simulink model "PLL_sim_a"  (R2020a)
settings: Solver=ode45  StartTime=0.0  StopTime=5  RelTol=1e-6  EnableMultiTasking=on
undefined symbols (not defined in the file): Cf, Kvco, R1, R2, Ts, VDD
libraries: msbPllFoundation x2
settings Model: Creator=nicolas  LastModifiedBy=svanico
settings SolverCC: SolverResetMethod=Robust
settings DataIOCC: LimitDataPoints=on  SaveFormat=Array  SignalLoggingSaveFormat=ModelDataLogs  ReturnWorkspaceOutputs=off
settings OptimizationCC: ExpressionDepthLimit=2147483647  LifeSpan=inf
settings DebuggingCC: UnderspecifiedInitializationDetection=Classic  MergeDetectMultiDrivingBlocksExec=none  SolverPrmCheckMsg=warning  FcnCallInpInsideContextMsg=warning  StateNameClashWarn=warning  SFUnexpectedBacktrackingDiag=warning  SFNoUnconditionalDefaultTransitionDiag=warning  SFExecutionAtInitializationDiag=none  ArithmeticOperatorsInVariantConditions=warning
settings HardwareCC: ProdBitPerPointer=32  ProdBitPerSizeT=32  ProdBitPerPtrDiffT=32  ProdLargestAtomicFloat=None  ProdIntDivRoundTo=Undefined  ProdEndianess=Unspecified  ProdWordSize=32  ProdHWDeviceType=32-bit Generic
settings ModelReferenceCC: EnableRefExpFcnMdlSchedulingChecks=off  PropagateSignalLabelsOutOfModel=off
settings SFSimCC: SimUseLocalCustomCode=off  CustomCodeUndefinedFunction=UseInterfaceOnly
settings RTWCC: RTWUseLocalCustomCode=off
settings CodeAppCC: StateflowObjectComments=on
settings GRTTargetCC: TargetLangStandard=C89/C90 (ANSI)  CombineOutputUpdateFcns=off  GRTInterface=on
settings ConfigComp: CovMetricSettings=dw  CovSaveCumulativeToWorkspaceVar=on  CovSaveSingleToWorkspaceVar=on  CovExternalEMLEnable=off

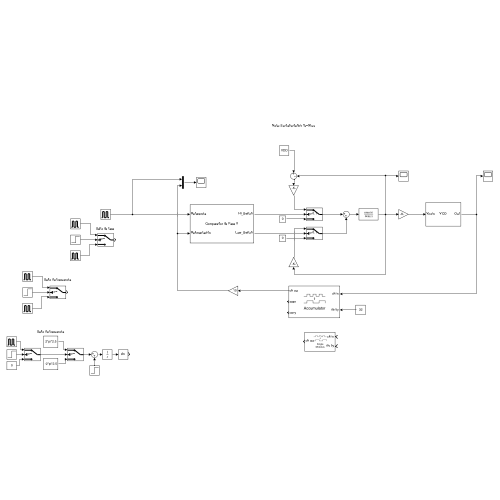
[thumbnail: Simulink's stored preview of the top-level diagram]
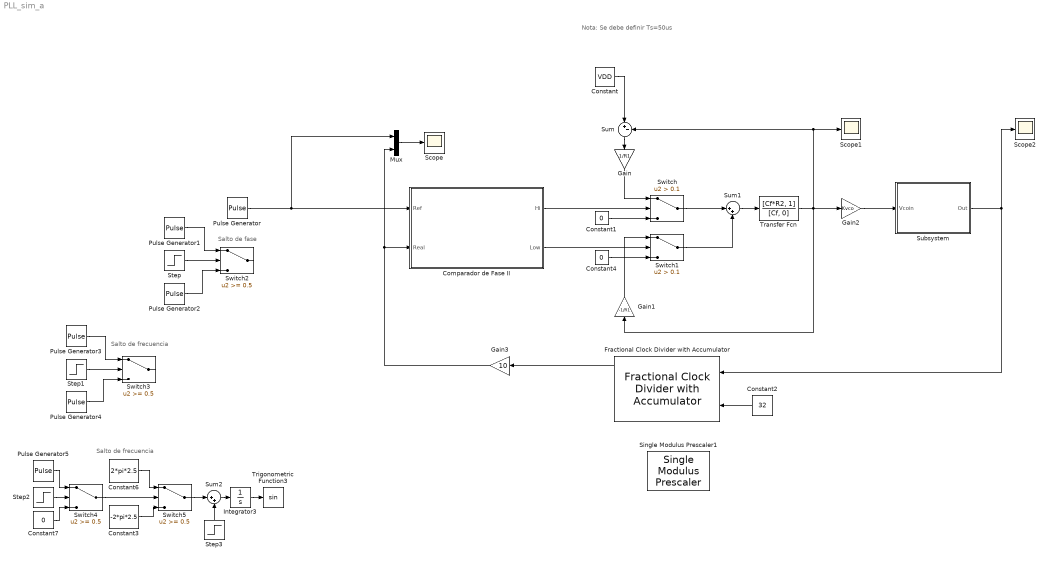
== system PLL_sim_a ==
  note: Nota: Se debe definir Ts=50us
  note: Salto de fase
  note: Salto de frecuencia
  note: Salto de frecuencia
  Comparador de Fase II : Subsystem  mask{Ts=Ts}
      mask Display:
      | disp('Comparador de Fase II')
      | port_label('input',1,'Referencia')
      | port_label('input',2,'Relimentación')
      | port_label('output',1,'Hi_Switch')
      | port_label('output',2,'Low_Switch')
  Constant : Constant  Value=VDD
  Constant1 : Constant  Value=0
  Constant2 : Constant  Value=32
  Constant3 : Constant  Value=-2*pi*2.5
  Constant4 : Constant  Value=0
  Constant6 : Constant  Value=2*pi*2.5
  Constant7 : Constant  Value=0
  Fractional Clock Divider with Accumulator : msbPllFoundation/Fractional Clock Divider with Accumulator  ExtraBuffer=on  NBuffer=1000
  Gain : Gain  Gain=1/R1
  Gain1 : Gain  Gain=-1/R1
  Gain2 : Gain  Gain=Kvco
  Gain3 : Gain  Gain=10
  Integrator3 : Integrator
  Mux : Mux  Inputs=2
  Pulse Generator : DiscretePulseGenerator  PulseType=Time based  Amplitude=10  Period=1/50  PulseWidth=50
  Pulse Generator1 : DiscretePulseGenerator  PulseType=Time based  Amplitude=10  Period=1/50  PulseWidth=50  PhaseDelay=1/400
  Pulse Generator2 : DiscretePulseGenerator  PulseType=Time based  Amplitude=10  Period=1/50  PulseWidth=50
  Pulse Generator3 : DiscretePulseGenerator  PulseType=Time based  Amplitude=10  Period=1/50  PulseWidth=50
  Pulse Generator4 : DiscretePulseGenerator  PulseType=Time based  Amplitude=10  Period=1/51  PulseWidth=50
  Pulse Generator5 : DiscretePulseGenerator  PulseType=Time based  Period=0.5  PulseWidth=50
  Scope : Scope
  Scope1 : Scope
  Scope2 : Scope
  Single Modulus Prescaler1 : msbPllFoundation/Single Modulus Prescaler  ExtraBuffer=off  NBuffer=1000
  Step : Step  Time=10/50  After=2  SampleTime=0
  Step1 : Step  Time=10/50  After=2  SampleTime=0
  Step2 : Step  Time=.5  After=2  SampleTime=0
  Step3 : Step  Time=0  After=2*pi*50  SampleTime=0
  Subsystem : Subsystem  mask{Ts=Ts}
      mask Display:
      | disp('VCO')
      | port_label('input',1,'Vcoin')
      | port_label('output',1,'Out')
  Sum : Sum  Inputs=|+-
  Sum1 : Sum  Inputs=|++
  Sum2 : Sum  Inputs=|++
  Switch : Switch  Criteria=u2 > Threshold  Threshold=0.1
  Switch1 : Switch  Criteria=u2 > Threshold  Threshold=0.1
  Switch{2..5} (4 alike) : Switch  Threshold=0.5
  Transfer Fcn : TransferFcn  Numerator=[Cf*R2, 1]  Denominator=[Cf, 0]
  Trigonometric Function3 : Trigonometry
  wires:
  Gain2/1 -> Subsystem/1(Vcoin)
  Sum1/1 -> Transfer Fcn/1
  Switch1/1 -> Sum1/2
  Constant/1 -> Sum/1
  Constant2/1 -> Fractional Clock Divider with Accumulator/2
  Constant1/1 -> Switch/3
  Switch/1 -> Sum1/1
  Gain/1 -> Switch/1
  Sum/1 -> Gain/1
  Comparador de Fase II/2(Low) -> Switch1/2
  Comparador de Fase II/1(Hi) -> Switch/2
  Subsystem/1(Out) -> Fractional Clock Divider with Accumulator/1, Scope2/1
  Fractional Clock Divider with Accumulator/1 -> Gain3/1
  Pulse Generator/1 -> Mux/1, Comparador de Fase II/1(Ref)
  Gain3/1 -> Mux/2, Comparador de Fase II/2(Real)
  Transfer Fcn/1 -> Gain1/1, Sum/2, Scope1/1, Gain2/1
  Pulse Generator2/1 -> Switch2/3
  Step/1 -> Switch2/2
  Pulse Generator1/1 -> Switch2/1
  Pulse Generator4/1 -> Switch3/3
  Step1/1 -> Switch3/2
  Pulse Generator3/1 -> Switch3/1
  Constant3/1 -> Switch5/3
  Step2/1 -> Switch4/2
  Switch5/1 -> Sum2/1
  Pulse Generator5/1 -> Switch4/1
  Constant6/1 -> Switch5/1
  Constant7/1 -> Switch4/3
  Step3/1 -> Sum2/2
  Sum2/1 -> Integrator3/1
  Integrator3/1 -> Trigonometric Function3/1
  Switch4/1 -> Switch5/2
  Gain1/1 -> Switch1/1
  Constant4/1 -> Switch1/3
  Mux/1 -> Scope/1

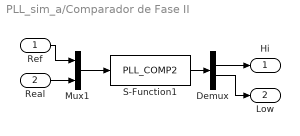
== system PLL_sim_a/Comparador de Fase II ==
  Ref : Inport
  Real : Inport  Port=2
  Demux : Demux
  Mux1 : Mux  Inputs=2
  S-Function1 : S-Function  FunctionName=PLL_COMP2  Parameters=Ts  SFunctionDeploymentMode=off  EnableBusSupport=off
  Hi : Outport
  Low : Outport  Port=2
  wires:
  Mux1/1 -> S-Function1/1
  S-Function1/1 -> Demux/1
  Ref/1 -> Mux1/1
  Demux/2 -> Hi/1
  Demux/3 -> Low/1
  Real/1 -> Mux1/2

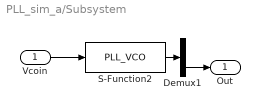
== system PLL_sim_a/Subsystem ==
  Vcoin : Inport
  Demux1 : Demux  Outputs=2
  S-Function2 : S-Function  FunctionName=PLL_VCO  Parameters=Ts  SFunctionDeploymentMode=off  EnableBusSupport=off
  Out : Outport
  wires:
  S-Function2/1 -> Demux1/1
  Vcoin/1 -> S-Function2/1
  Demux1/2 -> Out/1
